simulink model "yin_2009"  (R2016a)
settings: Solver=VariableStepAuto  StartTime=0.0  StopTime=2.15  RelTol=1e-3
values from neighbouring files (symbols this model uses):
  alpha = 0.9    [param.mat]
  g = 9.8    [param.mat]
  J_w = 0.5    [param.mat]
  M = 360    [param.mat]
  r = 0.22    [param.mat]
  t_m = 0.001    [param.mat]
  taw1 = 0.02    [param.mat]
  taw2 = 0.02    [param.mat]
libraries: simulink x1
settings Model: Creator=M  LastModifiedBy=M

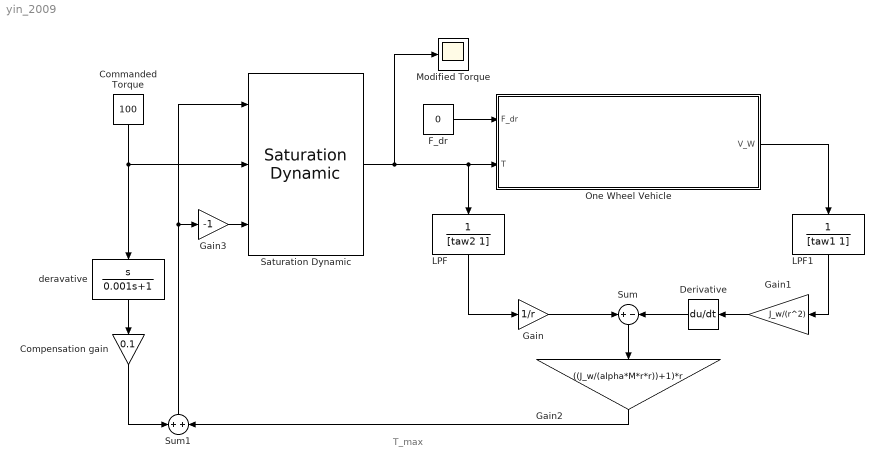
== system yin_2009 ==
  note: T_max
  Commanded Torque : Constant  Value=100
  Compensation gain : Gain  Gain=0.1
  Derivative : Derivative
  F_dr : Constant  Value=0
  Gain : Gain  Gain=1/r
  Gain1 : Gain  Gain=J_w/(r^2)
  Gain2 : Gain  Gain=((J_w/(alpha*M*r*r))+1)*r
  Gain3 : Gain  Gain=-1
  LPF : TransferFcn  Denominator=[taw2 1]
  LPF1 : TransferFcn  Denominator=[taw1 1]
  Modified Torque : Scope
  One Wheel Vehicle : Subsystem
  Saturation Dynamic : simulink/Discontinuities/Saturation Dynamic  OutMin=[]  OutMax=[]  OutDataTypeStr=Inherit: Same as second input  OutDataType=fixdt(1, 16)  OutScaling=2^-10  DoSatur=off
  Sum : Sum  Inputs=+|-
  Sum1 : Sum  Inputs=+|+
  deravative : TransferFcn  Numerator=[1 0]  Denominator=[0.001 1]
  wires:
  One Wheel Vehicle/1(V_W) -> LPF1/1
  Saturation Dynamic/1 -> Modified Torque/1, LPF/1, One Wheel Vehicle/2(T)
  LPF/1 -> Gain/1
  Gain1/1 -> Derivative/1
  LPF1/1 -> Gain1/1
  Derivative/1 -> Sum/2
  Gain/1 -> Sum/1
  Sum/1 -> Gain2/1
  Gain3/1 -> Saturation Dynamic/3
  F_dr/1 -> One Wheel Vehicle/1(F_dr)
  Sum1/1 -> Gain3/1, Saturation Dynamic/1
  Gain2/1 -> Sum1/2
  deravative/1 -> Compensation gain/1
  Compensation gain/1 -> Sum1/1
  Commanded Torque/1 -> deravative/1, Saturation Dynamic/2

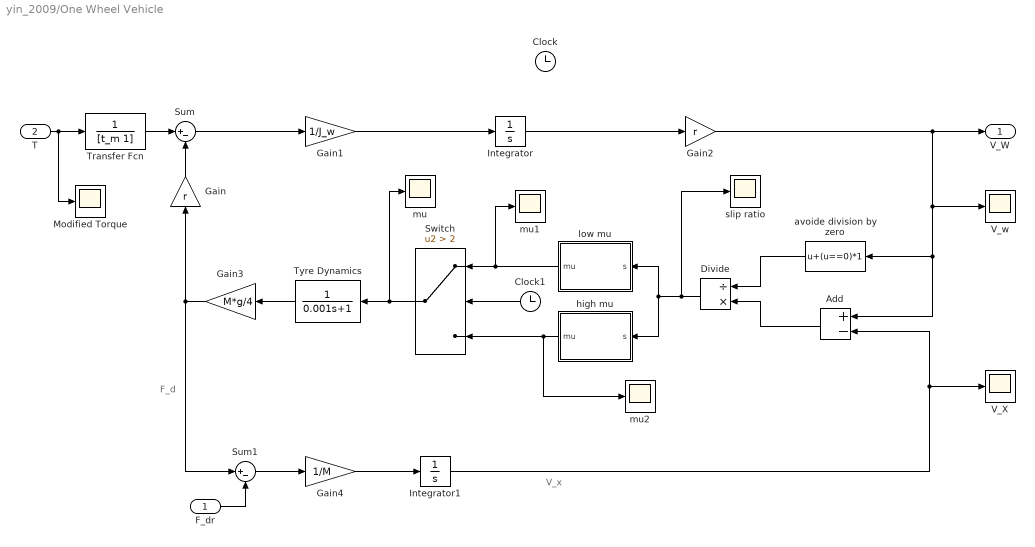
== system yin_2009/One Wheel Vehicle ==
  note: F_d
  note: V_x
  F_dr : Inport
  T : Inport  Port=2
  Add : Sum  Inputs=+-
  Clock : Clock
  Clock1 : Clock
  Divide : Product  Inputs=/*
  Gain : Gain  Gain=r
  Gain1 : Gain  Gain=1/J_w
  Gain2 : Gain  Gain=r
  Gain3 : Gain  Gain=M*g/4
  Gain4 : Gain  Gain=1/M
  Integrator : Integrator
  Integrator1 : Integrator
  Modified Torque : Scope
  Sum : Sum  Inputs=|+-
  Sum1 : Sum  Inputs=|+-
  Switch : Switch  Criteria=u2 > Threshold  Threshold=2  ZeroCross=off
  Transfer Fcn : TransferFcn  Denominator=[t_m 1]
  Tyre Dynamics : TransferFcn  Denominator=[0.001 1]
  V_X : Scope
  V_w : Scope
  avoide division by zero : MATLABFcn  MATLABFcn=u+(u==0)*1
  high mu : MATLAB Function  TreatAsAtomicUnit=on
  low mu : MATLAB Function  TreatAsAtomicUnit=on
  mu : Scope
  mu1 : Scope
  mu2 : Scope
  slip ratio : Scope
  V_W : Outport
  wires:
  Gain/1 -> Sum/2
  Transfer Fcn/1 -> Sum/1
  Sum/1 -> Gain1/1
  Gain1/1 -> Integrator/1
  Integrator/1 -> Gain2/1
  Tyre Dynamics/1 -> Gain3/1
  Gain3/1 -> Gain/1, Sum1/1
  Sum1/1 -> Gain4/1
  Gain4/1 -> Integrator1/1
  T/1 -> Modified Torque/1, Transfer Fcn/1
  F_dr/1 -> Sum1/2
  Switch/1 -> mu/1, Tyre Dynamics/1
  low mu/1(mu) -> mu1/1, Switch/1
  high mu/1(mu) -> Switch/3, mu2/1
  Integrator1/1 -> V_X/1, Add/2
  Add/1 -> Divide/2
  Gain2/1 -> V_W/1, Add/1, avoide division by zero/1, V_w/1
  avoide division by zero/1 -> Divide/1
  Divide/1 -> slip ratio/1, high mu/1(s), low mu/1(s)
  Clock1/1 -> Switch/2

== matlab function yin_2009/One Wheel Vehicle/high mu ==
  data: s input; mu output
function mu = fcn(s)

mu = sin(1.9 * atan(  10*s-0.97*(10*s-atan( 10*s )))  );

== matlab function yin_2009/One Wheel Vehicle/low mu ==
  data: s input; mu output
function mu = fcn(s)

mu = 0.3*sin(2 * atan(  5*s-1*(5*s-atan( 5*s )))  );
